simulink model "SecRwRtStRclCmdSrvCal"  (R2018b)
settings: Solver=FixedStepDiscrete  StartTime=0.0  StopTime=10.0  FixedStep=0.01  RelTol=1e-3
undefined symbols (not defined in the file or in its folder): KeSMSwPosInvalidVal_Val, PowerMode1
settings Model: Creator=sn2xws  LastModifiedBy=sn2xws
settings Model: ModifiedHistory=|
  | 2024.5.6
  | 557 新增零重力电机
settings DataIOCC: SaveFormat=StructureWithTime
settings OptimizationCC: DefaultParameterBehavior=Inlined  EnhancedBackFolding=on  PassReuseOutputArgsAs=Individual arguments  ZeroExternalMemoryAtStartup=off  ZeroInternalMemoryAtStartup=off  OptimizeBlockOrder=speed  DifferentSizesBufferReuse=on  OptimizationCustomize=off
settings DebuggingCC: ParameterTunabilityLossMsg=error
settings ModelReferenceCC: ModelReferenceNumInstancesAllowed=Single
settings SFSimCC: MATLABDynamicMemAlloc=off
settings RTWCC: SystemTargetFile=autosar.tlc  GenCodeOnly=on  TemplateMakefile=ert_default_tmf  Description=AUTOSAR  GenerateReport=on  IncludeHyperlinkInReport=on  LaunchReport=on  GenerateTraceInfo=on  GenerateTraceReport=on  GenerateTraceReportSl=on  GenerateTraceReportSf=on  GenerateTraceReportEml=on  GenerateCodeMetricsReport=on
settings CodeAppCC: ForceParamTrailComments=on  IgnoreCustomStorageClasses=off  OperatorAnnotations=on  SimulinkDataObjDesc=on  SFDataObjDesc=on  InsertBlockDesc=on
settings STFCustomTargetCC: TargetLangStandard=C99 (ISO)  MultiwordLength=256  ParMdlRefBuildCompliant=on  CompOptLevelCompliant=on  IncludeMdlTerminateFcn=off  CombineOutputUpdateFcns=on  SuppressErrorStatus=on  ERTCustomFileBanners=on  SupportNonFinite=off  SupportComplex=off  SupportContinuousTime=off  SupportNonInlinedSFcns=off  RemoveResetFunc=on  MATLABClassNameForMDSCustomization=Simulink.SoftwareTarget.ERTCustomization  AutosarCompliant=on  UseToolchainInfoCompliant=on  LookupTableObjectStructAxisOrder=2,1,3,4,...  LUTObjectStructOrderEvenSpacing=Size,Table,Breakpoints  SystemTargetFile=autosar.tlc
settings ERTTargetCC: TargetLangStandard=C99 (ISO)  ConcurrentExecutionCompliant=off  IncludeMdlTerminateFcn=off  SuppressErrorStatus=on  SupportNonFinite=off  SupportComplex=off  ModelStepFunctionPrototypeControlCompliant=off  CPPClassGenCompliant=off  AutosarCompliant=on  LookupTableObjectStructAxisOrder=2,1,3,4,...  LUTObjectStructOrderEvenSpacing=Size,Table,Breakpoints  InlinedParameterPlacement=NonHierarchical  ERTCustomFileTemplate=example_file_process.tlc  ERTFilePackagingFormat=Compact

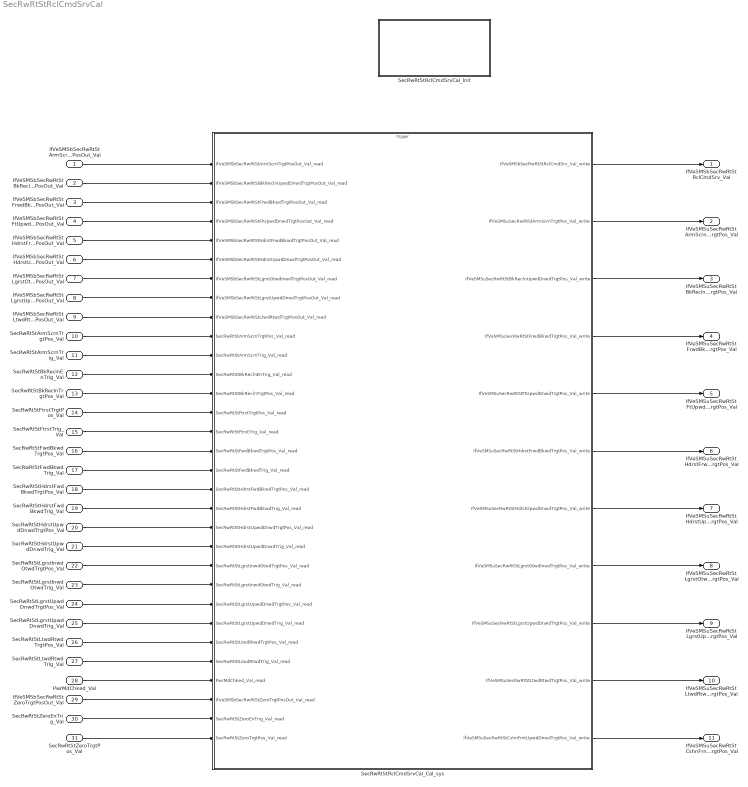
== system SecRwRtStRclCmdSrvCal ==
  IfVeSMSbSecRwRtStArmScrnTrgtPosOut_Val : Inport  OutDataTypeStr=boolean  PortDimensions=1
  IfVeSMSbSecRwRtStBkReclnUpwdDnwdTrgtPosOut_Val : Inport  Port=2  OutDataTypeStr=boolean  PortDimensions=1
  IfVeSMSbSecRwRtStFrwdBkwdTrgtPosOut_Val : Inport  Port=3  OutDataTypeStr=boolean  PortDimensions=1
  IfVeSMSbSecRwRtStFtUpwdDnwdTrgtPosOut_Val : Inport  Port=4  OutDataTypeStr=boolean  PortDimensions=1
  IfVeSMSbSecRwRtStHdrstFrwdBkwdTrgtPosOut_Val : Inport  Port=5  OutDataTypeStr=boolean  PortDimensions=1
  IfVeSMSbSecRwRtStHdrstUpwdDnwdTrgtPosOut_Val : Inport  Port=6  OutDataTypeStr=boolean  PortDimensions=1
  IfVeSMSbSecRwRtStLgrstOtwdInwdTrgtPosOut_Val : Inport  Port=7  OutDataTypeStr=boolean  PortDimensions=1
  IfVeSMSbSecRwRtStLgrstUpwdDnwdTrgtPosOut_Val : Inport  Port=8  OutDataTypeStr=boolean  PortDimensions=1
  IfVeSMSbSecRwRtStLtwdRtwdTrgtPosOut_Val : Inport  Port=9  OutDataTypeStr=boolean  PortDimensions=1
  SecRwRtStArmScrnTrgtPos_Val : Inport  Port=10  OutDataTypeStr=uint16  PortDimensions=1
  SecRwRtStArmScrnTrig_Val : Inport  Port=11  OutDataTypeStr=boolean  PortDimensions=1
  SecRwRtStBkReclnEnTrig_Val : Inport  Port=12  OutDataTypeStr=boolean  PortDimensions=1
  SecRwRtStBkReclnTrgtPos_Val : Inport  Port=13  OutDataTypeStr=uint16  PortDimensions=1
  SecRwRtStFtrstTrgtPos_Val : Inport  Port=14  OutDataTypeStr=uint16  PortDimensions=1
  SecRwRtStFtrstTrig_Val : Inport  Port=15  OutDataTypeStr=boolean  PortDimensions=1
  SecRwRtStFwdBkwdTrgtPos_Val : Inport  Port=16  OutDataTypeStr=uint16  PortDimensions=1
  SecRwRtStFwdBkwdTrig_Val : Inport  Port=17  OutDataTypeStr=boolean  PortDimensions=1
  SecRwRtStHdrstFwdBkwdTrgtPos_Val : Inport  Port=18  OutDataTypeStr=uint16  PortDimensions=1
  SecRwRtStHdrstFwdBkwdTrig_Val : Inport  Port=19  OutDataTypeStr=boolean  PortDimensions=1
  SecRwRtStHdrstUpwdDnwdTrgtPos_Val : Inport  Port=20  OutDataTypeStr=uint16  PortDimensions=1
  SecRwRtStHdrstUpwdDnwdTrig_Val : Inport  Port=21  OutDataTypeStr=boolean  PortDimensions=1
  SecRwRtStLgrstInwdOtwdTrgtPos_Val : Inport  Port=22  OutDataTypeStr=uint16  PortDimensions=1
  SecRwRtStLgrstInwdOtwdTrig_Val : Inport  Port=23  OutDataTypeStr=boolean  PortDimensions=1
  SecRwRtStLgrstUpwdDnwdTrgtPos_Val : Inport  Port=24  OutDataTypeStr=uint16  PortDimensions=1
  SecRwRtStLgrstUpwdDnwdTrig_Val : Inport  Port=25  OutDataTypeStr=boolean  PortDimensions=1
  SecRwRtStLtwdRtwdTrgtPos_Val : Inport  Port=26  OutDataTypeStr=uint16  PortDimensions=1
  SecRwRtStLtwdRtwdTrig_Val : Inport  Port=27  OutDataTypeStr=boolean  PortDimensions=1
  PwrMdChked_Val : Inport  Port=28  OutDataTypeStr=Enum: PowerMode1  PortDimensions=1
  IfVeSMSbSecRwRtStZeroTrgtPosOut_Val : Inport  Port=29  OutDataTypeStr=boolean  PortDimensions=1
  SecRwRtStZeroEnTrig_Val : Inport  Port=30  OutDataTypeStr=boolean  PortDimensions=1
  SecRwRtStZeroTrgtPos_Val : Inport  Port=31  OutDataTypeStr=uint16  PortDimensions=1
  SecRwRtStRclCmdSrvCal_Cal_sys : Subsystem
  SecRwRtStRclCmdSrvCal_Init : Subsystem
  IfVeSMSbSecRwRtStRclCmdSrv_Val : Outport  OutDataTypeStr=boolean  PortDimensions=1
  IfVeSMSuSecRwRtStArmScrnTrgtPos_Val : Outport  Port=2  OutDataTypeStr=uint16  PortDimensions=1
  IfVeSMSuSecRwRtStBkReclnUpwdDnwdTrgtPos_Val : Outport  Port=3  OutDataTypeStr=uint16  PortDimensions=1
  IfVeSMSuSecRwRtStFrwdBkwdTrgtPos_Val : Outport  Port=4  OutDataTypeStr=uint16  PortDimensions=1
  IfVeSMSuSecRwRtStFtUpwdDnwdTrgtPos_Val : Outport  Port=5  OutDataTypeStr=uint16  PortDimensions=1
  IfVeSMSuSecRwRtStHdrstFrwdBkwdTrgtPos_Val : Outport  Port=6  OutDataTypeStr=uint16  PortDimensions=1
  IfVeSMSuSecRwRtStHdrstUpwdDnwdTrgtPos_Val : Outport  Port=7  OutDataTypeStr=uint16  PortDimensions=1
  IfVeSMSuSecRwRtStLgrstOtwdInwdTrgtPos_Val : Outport  Port=8  OutDataTypeStr=uint16  PortDimensions=1
  IfVeSMSuSecRwRtStLgrstUpwdDnwdTrgtPos_Val : Outport  Port=9  OutDataTypeStr=uint16  PortDimensions=1
  IfVeSMSuSecRwRtStLtwdRtwdTrgtPos_Val : Outport  Port=10  OutDataTypeStr=uint16  PortDimensions=1
  IfVeSMSuSecRwRtStCshnFrntUpwdDnwdTrgtPos_Val : Outport  Port=11  OutDataTypeStr=uint16  PortDimensions=1
  wires:
  IfVeSMSbSecRwRtStArmScrnTrgtPosOut_Val/1 -> SecRwRtStRclCmdSrvCal_Cal_sys/1(IfVeSMSbSecRwRtStArmScrnTrgtPosOut_Val_read)
  IfVeSMSbSecRwRtStBkReclnUpwdDnwdTrgtPosOut_Val/1 -> SecRwRtStRclCmdSrvCal_Cal_sys/2(IfVeSMSbSecRwRtStBkReclnUpwdDnwdTrgtPosOut_Val_read)
  IfVeSMSbSecRwRtStFrwdBkwdTrgtPosOut_Val/1 -> SecRwRtStRclCmdSrvCal_Cal_sys/3(IfVeSMSbSecRwRtStFrwdBkwdTrgtPosOut_Val_read)
  IfVeSMSbSecRwRtStFtUpwdDnwdTrgtPosOut_Val/1 -> SecRwRtStRclCmdSrvCal_Cal_sys/4(IfVeSMSbSecRwRtStFtUpwdDnwdTrgtPosOut_Val_read)
  IfVeSMSbSecRwRtStHdrstFrwdBkwdTrgtPosOut_Val/1 -> SecRwRtStRclCmdSrvCal_Cal_sys/5(IfVeSMSbSecRwRtStHdrstFrwdBkwdTrgtPosOut_Val_read)
  IfVeSMSbSecRwRtStHdrstUpwdDnwdTrgtPosOut_Val/1 -> SecRwRtStRclCmdSrvCal_Cal_sys/6(IfVeSMSbSecRwRtStHdrstUpwdDnwdTrgtPosOut_Val_read)
  IfVeSMSbSecRwRtStLgrstOtwdInwdTrgtPosOut_Val/1 -> SecRwRtStRclCmdSrvCal_Cal_sys/7(IfVeSMSbSecRwRtStLgrstOtwdInwdTrgtPosOut_Val_read)
  IfVeSMSbSecRwRtStLgrstUpwdDnwdTrgtPosOut_Val/1 -> SecRwRtStRclCmdSrvCal_Cal_sys/8(IfVeSMSbSecRwRtStLgrstUpwdDnwdTrgtPosOut_Val_read)
  IfVeSMSbSecRwRtStLtwdRtwdTrgtPosOut_Val/1 -> SecRwRtStRclCmdSrvCal_Cal_sys/9(IfVeSMSbSecRwRtStLtwdRtwdTrgtPosOut_Val_read)
  SecRwRtStArmScrnTrgtPos_Val/1 -> SecRwRtStRclCmdSrvCal_Cal_sys/10(SecRwRtStArmScrnTrgtPos_Val_read)
  SecRwRtStArmScrnTrig_Val/1 -> SecRwRtStRclCmdSrvCal_Cal_sys/11(SecRwRtStArmScrnTrig_Val_read)
  SecRwRtStBkReclnEnTrig_Val/1 -> SecRwRtStRclCmdSrvCal_Cal_sys/12(SecRwRtStBkReclnEnTrig_Val_read)
  SecRwRtStBkReclnTrgtPos_Val/1 -> SecRwRtStRclCmdSrvCal_Cal_sys/13(SecRwRtStBkReclnTrgtPos_Val_read)
  SecRwRtStFtrstTrgtPos_Val/1 -> SecRwRtStRclCmdSrvCal_Cal_sys/14(SecRwRtStFtrstTrgtPos_Val_read)
  SecRwRtStFtrstTrig_Val/1 -> SecRwRtStRclCmdSrvCal_Cal_sys/15(SecRwRtStFtrstTrig_Val_read)
  SecRwRtStFwdBkwdTrgtPos_Val/1 -> SecRwRtStRclCmdSrvCal_Cal_sys/16(SecRwRtStFwdBkwdTrgtPos_Val_read)
  SecRwRtStFwdBkwdTrig_Val/1 -> SecRwRtStRclCmdSrvCal_Cal_sys/17(SecRwRtStFwdBkwdTrig_Val_read)
  SecRwRtStHdrstFwdBkwdTrgtPos_Val/1 -> SecRwRtStRclCmdSrvCal_Cal_sys/18(SecRwRtStHdrstFwdBkwdTrgtPos_Val_read)
  SecRwRtStHdrstFwdBkwdTrig_Val/1 -> SecRwRtStRclCmdSrvCal_Cal_sys/19(SecRwRtStHdrstFwdBkwdTrig_Val_read)
  SecRwRtStHdrstUpwdDnwdTrgtPos_Val/1 -> SecRwRtStRclCmdSrvCal_Cal_sys/20(SecRwRtStHdrstUpwdDnwdTrgtPos_Val_read)
  SecRwRtStHdrstUpwdDnwdTrig_Val/1 -> SecRwRtStRclCmdSrvCal_Cal_sys/21(SecRwRtStHdrstUpwdDnwdTrig_Val_read)
  SecRwRtStLgrstInwdOtwdTrgtPos_Val/1 -> SecRwRtStRclCmdSrvCal_Cal_sys/22(SecRwRtStLgrstInwdOtwdTrgtPos_Val_read)
  SecRwRtStLgrstInwdOtwdTrig_Val/1 -> SecRwRtStRclCmdSrvCal_Cal_sys/23(SecRwRtStLgrstInwdOtwdTrig_Val_read)
  SecRwRtStLgrstUpwdDnwdTrgtPos_Val/1 -> SecRwRtStRclCmdSrvCal_Cal_sys/24(SecRwRtStLgrstUpwdDnwdTrgtPos_Val_read)
  SecRwRtStLgrstUpwdDnwdTrig_Val/1 -> SecRwRtStRclCmdSrvCal_Cal_sys/25(SecRwRtStLgrstUpwdDnwdTrig_Val_read)
  SecRwRtStLtwdRtwdTrgtPos_Val/1 -> SecRwRtStRclCmdSrvCal_Cal_sys/26(SecRwRtStLtwdRtwdTrgtPos_Val_read)
  SecRwRtStLtwdRtwdTrig_Val/1 -> SecRwRtStRclCmdSrvCal_Cal_sys/27(SecRwRtStLtwdRtwdTrig_Val_read)
  SecRwRtStRclCmdSrvCal_Cal_sys/1(IfVeSMSbSecRwRtStRclCmdSrv_Val_write) -> IfVeSMSbSecRwRtStRclCmdSrv_Val/1
  SecRwRtStRclCmdSrvCal_Cal_sys/2(IfVeSMSuSecRwRtStArmScrnTrgtPos_Val_write) -> IfVeSMSuSecRwRtStArmScrnTrgtPos_Val/1
  SecRwRtStRclCmdSrvCal_Cal_sys/3(IfVeSMSuSecRwRtStBkReclnUpwdDnwdTrgtPos_Val_write) -> IfVeSMSuSecRwRtStBkReclnUpwdDnwdTrgtPos_Val/1
  SecRwRtStRclCmdSrvCal_Cal_sys/4(IfVeSMSuSecRwRtStFrwdBkwdTrgtPos_Val_write) -> IfVeSMSuSecRwRtStFrwdBkwdTrgtPos_Val/1
  SecRwRtStRclCmdSrvCal_Cal_sys/5(IfVeSMSuSecRwRtStFtUpwdDnwdTrgtPos_Val_write) -> IfVeSMSuSecRwRtStFtUpwdDnwdTrgtPos_Val/1
  SecRwRtStRclCmdSrvCal_Cal_sys/6(IfVeSMSuSecRwRtStHdrstFrwdBkwdTrgtPos_Val_write) -> IfVeSMSuSecRwRtStHdrstFrwdBkwdTrgtPos_Val/1
  SecRwRtStRclCmdSrvCal_Cal_sys/7(IfVeSMSuSecRwRtStHdrstUpwdDnwdTrgtPos_Val_write) -> IfVeSMSuSecRwRtStHdrstUpwdDnwdTrgtPos_Val/1
  SecRwRtStRclCmdSrvCal_Cal_sys/8(IfVeSMSuSecRwRtStLgrstOtwdInwdTrgtPos_Val_write) -> IfVeSMSuSecRwRtStLgrstOtwdInwdTrgtPos_Val/1
  SecRwRtStRclCmdSrvCal_Cal_sys/9(IfVeSMSuSecRwRtStLgrstUpwdDnwdTrgtPos_Val_write) -> IfVeSMSuSecRwRtStLgrstUpwdDnwdTrgtPos_Val/1
  SecRwRtStRclCmdSrvCal_Cal_sys/10(IfVeSMSuSecRwRtStLtwdRtwdTrgtPos_Val_write) -> IfVeSMSuSecRwRtStLtwdRtwdTrgtPos_Val/1
  PwrMdChked_Val/1 -> SecRwRtStRclCmdSrvCal_Cal_sys/28(PwrMdChked_Val_read)
  IfVeSMSbSecRwRtStZeroTrgtPosOut_Val/1 -> SecRwRtStRclCmdSrvCal_Cal_sys/29(IfVeSMSbSecRwRtStZeroTrgtPosOut_Val_read)
  SecRwRtStZeroEnTrig_Val/1 -> SecRwRtStRclCmdSrvCal_Cal_sys/30(SecRwRtStZeroEnTrig_Val_read)
  SecRwRtStZeroTrgtPos_Val/1 -> SecRwRtStRclCmdSrvCal_Cal_sys/31(SecRwRtStZeroTrgtPos_Val_read)
  SecRwRtStRclCmdSrvCal_Cal_sys/11(IfVeSMSuSecRwRtStCshnFrntUpwdDnwdTrgtPos_Val_write) -> IfVeSMSuSecRwRtStCshnFrntUpwdDnwdTrgtPos_Val/1

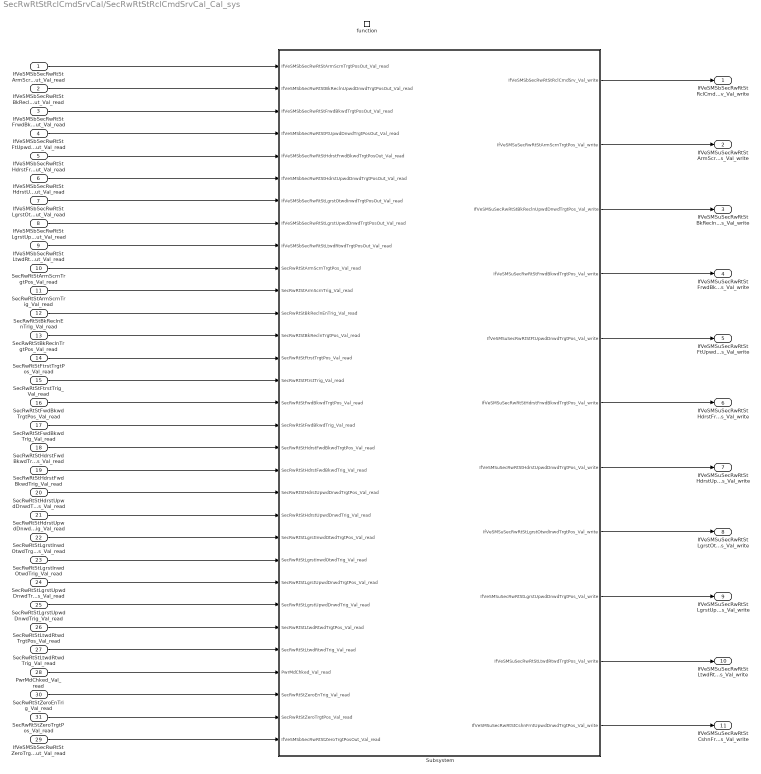
== system SecRwRtStRclCmdSrvCal/SecRwRtStRclCmdSrvCal_Cal_sys ==
  IfVeSMSbSecRwRtStArmScrnTrgtPosOut_Val_read : Inport
  IfVeSMSbSecRwRtStBkReclnUpwdDnwdTrgtPosOut_Val_read : Inport  Port=2
  IfVeSMSbSecRwRtStFrwdBkwdTrgtPosOut_Val_read : Inport  Port=3
  IfVeSMSbSecRwRtStFtUpwdDnwdTrgtPosOut_Val_read : Inport  Port=4
  IfVeSMSbSecRwRtStHdrstFrwdBkwdTrgtPosOut_Val_read : Inport  Port=5
  IfVeSMSbSecRwRtStHdrstUpwdDnwdTrgtPosOut_Val_read : Inport  Port=6
  IfVeSMSbSecRwRtStLgrstOtwdInwdTrgtPosOut_Val_read : Inport  Port=7
  IfVeSMSbSecRwRtStLgrstUpwdDnwdTrgtPosOut_Val_read : Inport  Port=8
  IfVeSMSbSecRwRtStLtwdRtwdTrgtPosOut_Val_read : Inport  Port=9
  SecRwRtStArmScrnTrgtPos_Val_read : Inport  Port=10
  SecRwRtStArmScrnTrig_Val_read : Inport  Port=11
  SecRwRtStBkReclnEnTrig_Val_read : Inport  Port=12
  SecRwRtStBkReclnTrgtPos_Val_read : Inport  Port=13
  SecRwRtStFtrstTrgtPos_Val_read : Inport  Port=14
  SecRwRtStFtrstTrig_Val_read : Inport  Port=15
  SecRwRtStFwdBkwdTrgtPos_Val_read : Inport  Port=16
  SecRwRtStFwdBkwdTrig_Val_read : Inport  Port=17
  SecRwRtStHdrstFwdBkwdTrgtPos_Val_read : Inport  Port=18
  SecRwRtStHdrstFwdBkwdTrig_Val_read : Inport  Port=19
  SecRwRtStHdrstUpwdDnwdTrgtPos_Val_read : Inport  Port=20
  SecRwRtStHdrstUpwdDnwdTrig_Val_read : Inport  Port=21
  SecRwRtStLgrstInwdOtwdTrgtPos_Val_read : Inport  Port=22
  SecRwRtStLgrstInwdOtwdTrig_Val_read : Inport  Port=23
  SecRwRtStLgrstUpwdDnwdTrgtPos_Val_read : Inport  Port=24
  SecRwRtStLgrstUpwdDnwdTrig_Val_read : Inport  Port=25
  SecRwRtStLtwdRtwdTrgtPos_Val_read : Inport  Port=26
  SecRwRtStLtwdRtwdTrig_Val_read : Inport  Port=27
  PwrMdChked_Val_read : Inport  Port=28
  IfVeSMSbSecRwRtStZeroTrgtPosOut_Val_read : Inport  Port=29
  SecRwRtStZeroEnTrig_Val_read : Inport  Port=30
  SecRwRtStZeroTrgtPos_Val_read : Inport  Port=31
  function : TriggerPort  TriggerType=function-call  IsSimulinkFunction=on  FunctionName=SecRwRtStRclCmdSrvCal_Cal  VariantControl=(inherit)
  Subsystem : Subsystem
  IfVeSMSbSecRwRtStRclCmdSrv_Val_write : Outport
      settings: EnsureOutportIsVirtual=on
  IfVeSMSuSecRwRtStArmScrnTrgtPos_Val_write : Outport  Port=2
      settings: EnsureOutportIsVirtual=on
  IfVeSMSuSecRwRtStBkReclnUpwdDnwdTrgtPos_Val_write : Outport  Port=3
      settings: EnsureOutportIsVirtual=on
  IfVeSMSuSecRwRtStFrwdBkwdTrgtPos_Val_write : Outport  Port=4
      settings: EnsureOutportIsVirtual=on
  IfVeSMSuSecRwRtStFtUpwdDnwdTrgtPos_Val_write : Outport  Port=5
      settings: EnsureOutportIsVirtual=on
  IfVeSMSuSecRwRtStHdrstFrwdBkwdTrgtPos_Val_write : Outport  Port=6
      settings: EnsureOutportIsVirtual=on
  IfVeSMSuSecRwRtStHdrstUpwdDnwdTrgtPos_Val_write : Outport  Port=7
      settings: EnsureOutportIsVirtual=on
  IfVeSMSuSecRwRtStLgrstOtwdInwdTrgtPos_Val_write : Outport  Port=8
      settings: EnsureOutportIsVirtual=on
  IfVeSMSuSecRwRtStLgrstUpwdDnwdTrgtPos_Val_write : Outport  Port=9
      settings: EnsureOutportIsVirtual=on
  IfVeSMSuSecRwRtStLtwdRtwdTrgtPos_Val_write : Outport  Port=10
      settings: EnsureOutportIsVirtual=on
  IfVeSMSuSecRwRtStCshnFrntUpwdDnwdTrgtPos_Val_write : Outport  Port=11
      settings: EnsureOutportIsVirtual=on
  wires:
  SecRwRtStFwdBkwdTrgtPos_Val_read/1 -> Subsystem/16(SecRwRtStFwdBkwdTrgtPos_Val_read)
  SecRwRtStFwdBkwdTrig_Val_read/1 -> Subsystem/17(SecRwRtStFwdBkwdTrig_Val_read)
  SecRwRtStHdrstFwdBkwdTrgtPos_Val_read/1 -> Subsystem/18(SecRwRtStHdrstFwdBkwdTrgtPos_Val_read)
  SecRwRtStFtrstTrgtPos_Val_read/1 -> Subsystem/14(SecRwRtStFtrstTrgtPos_Val_read)
  SecRwRtStFtrstTrig_Val_read/1 -> Subsystem/15(SecRwRtStFtrstTrig_Val_read)
  SecRwRtStHdrstFwdBkwdTrig_Val_read/1 -> Subsystem/19(SecRwRtStHdrstFwdBkwdTrig_Val_read)
  SecRwRtStHdrstUpwdDnwdTrgtPos_Val_read/1 -> Subsystem/20(SecRwRtStHdrstUpwdDnwdTrgtPos_Val_read)
  SecRwRtStArmScrnTrig_Val_read/1 -> Subsystem/11(SecRwRtStArmScrnTrig_Val_read)
  SecRwRtStBkReclnEnTrig_Val_read/1 -> Subsystem/12(SecRwRtStBkReclnEnTrig_Val_read)
  SecRwRtStBkReclnTrgtPos_Val_read/1 -> Subsystem/13(SecRwRtStBkReclnTrgtPos_Val_read)
  SecRwRtStHdrstUpwdDnwdTrig_Val_read/1 -> Subsystem/21(SecRwRtStHdrstUpwdDnwdTrig_Val_read)
  SecRwRtStLgrstInwdOtwdTrgtPos_Val_read/1 -> Subsystem/22(SecRwRtStLgrstInwdOtwdTrgtPos_Val_read)
  SecRwRtStLgrstInwdOtwdTrig_Val_read/1 -> Subsystem/23(SecRwRtStLgrstInwdOtwdTrig_Val_read)
  IfVeSMSbSecRwRtStLtwdRtwdTrgtPosOut_Val_read/1 -> Subsystem/9(IfVeSMSbSecRwRtStLtwdRtwdTrgtPosOut_Val_read)
  SecRwRtStArmScrnTrgtPos_Val_read/1 -> Subsystem/10(SecRwRtStArmScrnTrgtPos_Val_read)
  SecRwRtStLgrstUpwdDnwdTrgtPos_Val_read/1 -> Subsystem/24(SecRwRtStLgrstUpwdDnwdTrgtPos_Val_read)
  SecRwRtStLgrstUpwdDnwdTrig_Val_read/1 -> Subsystem/25(SecRwRtStLgrstUpwdDnwdTrig_Val_read)
  IfVeSMSbSecRwRtStHdrstUpwdDnwdTrgtPosOut_Val_read/1 -> Subsystem/6(IfVeSMSbSecRwRtStHdrstUpwdDnwdTrgtPosOut_Val_read)
  IfVeSMSbSecRwRtStLgrstOtwdInwdTrgtPosOut_Val_read/1 -> Subsystem/7(IfVeSMSbSecRwRtStLgrstOtwdInwdTrgtPosOut_Val_read)
  IfVeSMSbSecRwRtStLgrstUpwdDnwdTrgtPosOut_Val_read/1 -> Subsystem/8(IfVeSMSbSecRwRtStLgrstUpwdDnwdTrgtPosOut_Val_read)
  SecRwRtStLtwdRtwdTrgtPos_Val_read/1 -> Subsystem/26(SecRwRtStLtwdRtwdTrgtPos_Val_read)
  SecRwRtStLtwdRtwdTrig_Val_read/1 -> Subsystem/27(SecRwRtStLtwdRtwdTrig_Val_read)
  IfVeSMSbSecRwRtStFtUpwdDnwdTrgtPosOut_Val_read/1 -> Subsystem/4(IfVeSMSbSecRwRtStFtUpwdDnwdTrgtPosOut_Val_read)
  IfVeSMSbSecRwRtStHdrstFrwdBkwdTrgtPosOut_Val_read/1 -> Subsystem/5(IfVeSMSbSecRwRtStHdrstFrwdBkwdTrgtPosOut_Val_read)
  IfVeSMSbSecRwRtStArmScrnTrgtPosOut_Val_read/1 -> Subsystem/1(IfVeSMSbSecRwRtStArmScrnTrgtPosOut_Val_read)
  IfVeSMSbSecRwRtStBkReclnUpwdDnwdTrgtPosOut_Val_read/1 -> Subsystem/2(IfVeSMSbSecRwRtStBkReclnUpwdDnwdTrgtPosOut_Val_read)
  IfVeSMSbSecRwRtStFrwdBkwdTrgtPosOut_Val_read/1 -> Subsystem/3(IfVeSMSbSecRwRtStFrwdBkwdTrgtPosOut_Val_read)
  Subsystem/1(IfVeSMSbSecRwRtStRclCmdSrv_Val_write) -> IfVeSMSbSecRwRtStRclCmdSrv_Val_write/1
  Subsystem/2(IfVeSMSuSecRwRtStArmScrnTrgtPos_Val_write) -> IfVeSMSuSecRwRtStArmScrnTrgtPos_Val_write/1
  Subsystem/3(IfVeSMSuSecRwRtStBkReclnUpwdDnwdTrgtPos_Val_write) -> IfVeSMSuSecRwRtStBkReclnUpwdDnwdTrgtPos_Val_write/1
  Subsystem/4(IfVeSMSuSecRwRtStFrwdBkwdTrgtPos_Val_write) -> IfVeSMSuSecRwRtStFrwdBkwdTrgtPos_Val_write/1
  Subsystem/5(IfVeSMSuSecRwRtStFtUpwdDnwdTrgtPos_Val_write) -> IfVeSMSuSecRwRtStFtUpwdDnwdTrgtPos_Val_write/1
  Subsystem/6(IfVeSMSuSecRwRtStHdrstFrwdBkwdTrgtPos_Val_write) -> IfVeSMSuSecRwRtStHdrstFrwdBkwdTrgtPos_Val_write/1
  Subsystem/7(IfVeSMSuSecRwRtStHdrstUpwdDnwdTrgtPos_Val_write) -> IfVeSMSuSecRwRtStHdrstUpwdDnwdTrgtPos_Val_write/1
  Subsystem/8(IfVeSMSuSecRwRtStLgrstOtwdInwdTrgtPos_Val_write) -> IfVeSMSuSecRwRtStLgrstOtwdInwdTrgtPos_Val_write/1
  Subsystem/9(IfVeSMSuSecRwRtStLgrstUpwdDnwdTrgtPos_Val_write) -> IfVeSMSuSecRwRtStLgrstUpwdDnwdTrgtPos_Val_write/1
  Subsystem/10(IfVeSMSuSecRwRtStLtwdRtwdTrgtPos_Val_write) -> IfVeSMSuSecRwRtStLtwdRtwdTrgtPos_Val_write/1
  PwrMdChked_Val_read/1 -> Subsystem/28(PwrMdChked_Val_read)
  IfVeSMSbSecRwRtStZeroTrgtPosOut_Val_read/1 -> Subsystem/31(IfVeSMSbSecRwRtStZeroTrgtPosOut_Val_read)
  Subsystem/11(IfVeSMSuSecRwRtStCshnFrntUpwdDnwdTrgtPos_Val_write) -> IfVeSMSuSecRwRtStCshnFrntUpwdDnwdTrgtPos_Val_write/1
  SecRwRtStZeroEnTrig_Val_read/1 -> Subsystem/29(SecRwRtStZeroEnTrig_Val_read)
  SecRwRtStZeroTrgtPos_Val_read/1 -> Subsystem/30(SecRwRtStZeroTrgtPos_Val_read)

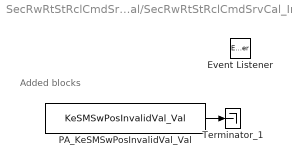
== system SecRwRtStRclCmdSrvCal/SecRwRtStRclCmdSrvCal_Init ==
  note: Added blocks
  Event Listener : EventListener  EventName=reset
  PA_KeSMSwPosInvalidVal_Val : Constant  Value=KeSMSwPosInvalidVal_Val
  Terminator_1 : Terminator
  wires:
  PA_KeSMSwPosInvalidVal_Val/1 -> Terminator_1/1

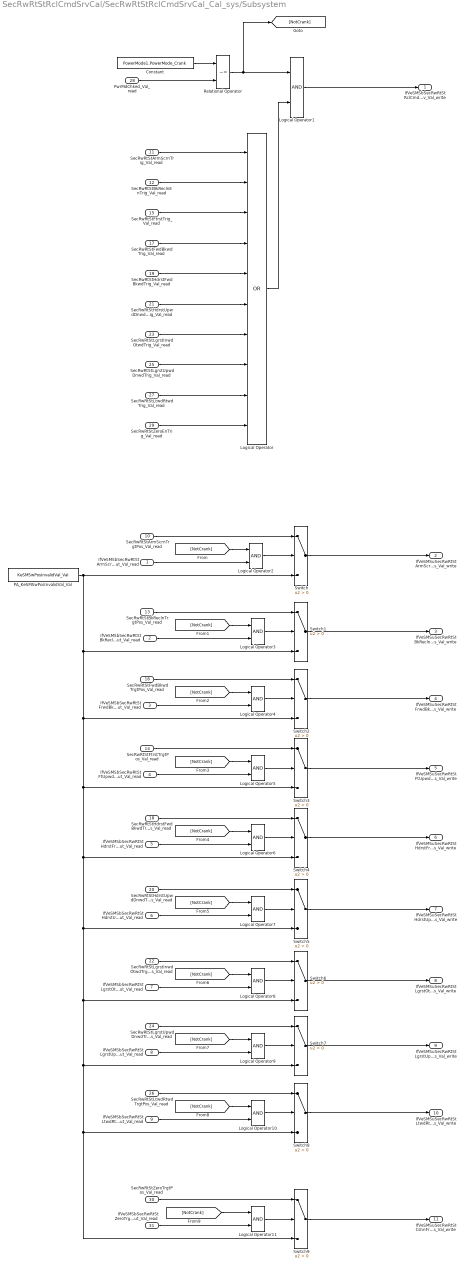
== system SecRwRtStRclCmdSrvCal/SecRwRtStRclCmdSrvCal_Cal_sys/Subsystem ==
  IfVeSMSbSecRwRtStArmScrnTrgtPosOut_Val_read : Inport
  IfVeSMSbSecRwRtStBkReclnUpwdDnwdTrgtPosOut_Val_read : Inport  Port=2
  IfVeSMSbSecRwRtStFrwdBkwdTrgtPosOut_Val_read : Inport  Port=3
  IfVeSMSbSecRwRtStFtUpwdDnwdTrgtPosOut_Val_read : Inport  Port=4
  IfVeSMSbSecRwRtStHdrstFrwdBkwdTrgtPosOut_Val_read : Inport  Port=5
  IfVeSMSbSecRwRtStHdrstUpwdDnwdTrgtPosOut_Val_read : Inport  Port=6
  IfVeSMSbSecRwRtStLgrstOtwdInwdTrgtPosOut_Val_read : Inport  Port=7
  IfVeSMSbSecRwRtStLgrstUpwdDnwdTrgtPosOut_Val_read : Inport  Port=8
  IfVeSMSbSecRwRtStLtwdRtwdTrgtPosOut_Val_read : Inport  Port=9
  SecRwRtStArmScrnTrgtPos_Val_read : Inport  Port=10
  SecRwRtStArmScrnTrig_Val_read : Inport  Port=11
  SecRwRtStBkReclnEnTrig_Val_read : Inport  Port=12
  SecRwRtStBkReclnTrgtPos_Val_read : Inport  Port=13
  SecRwRtStFtrstTrgtPos_Val_read : Inport  Port=14
  SecRwRtStFtrstTrig_Val_read : Inport  Port=15
  SecRwRtStFwdBkwdTrgtPos_Val_read : Inport  Port=16
  SecRwRtStFwdBkwdTrig_Val_read : Inport  Port=17
  SecRwRtStHdrstFwdBkwdTrgtPos_Val_read : Inport  Port=18
  SecRwRtStHdrstFwdBkwdTrig_Val_read : Inport  Port=19
  SecRwRtStHdrstUpwdDnwdTrgtPos_Val_read : Inport  Port=20
  SecRwRtStHdrstUpwdDnwdTrig_Val_read : Inport  Port=21
  SecRwRtStLgrstInwdOtwdTrgtPos_Val_read : Inport  Port=22
  SecRwRtStLgrstInwdOtwdTrig_Val_read : Inport  Port=23
  SecRwRtStLgrstUpwdDnwdTrgtPos_Val_read : Inport  Port=24
  SecRwRtStLgrstUpwdDnwdTrig_Val_read : Inport  Port=25
  SecRwRtStLtwdRtwdTrgtPos_Val_read : Inport  Port=26
  SecRwRtStLtwdRtwdTrig_Val_read : Inport  Port=27
  PwrMdChked_Val_read : Inport  Port=28
  SecRwRtStZeroEnTrig_Val_read : Inport  Port=29
  SecRwRtStZeroTrgtPos_Val_read : Inport  Port=30
  IfVeSMSbSecRwRtStZeroTrgtPosOut_Val_read : Inport  Port=31
  Constant : Constant  Value=PowerMode1.PowerMode_Crank  OutDataTypeStr=Enum: PowerMode1
  Logical Operator : Logic  Operator=OR  Inputs=10  AllPortsSameDT=off  OutDataTypeStr=boolean
  Logical Operator{1..11} (11 alike) : Logic  AllPortsSameDT=off  OutDataTypeStr=boolean
  PA_KeSMSwPosInvalidVal_Val : Constant  Value=KeSMSwPosInvalidVal_Val
  Relational Operator : RelationalOperator  Operator=~=  OutDataTypeStr=boolean  RndMeth=Simplest
  Switch{,1..9} (10 alike) : Switch  Criteria=u2 > Threshold
  IfVeSMSbSecRwRtStRclCmdSrv_Val_write : Outport
      settings: EnsureOutportIsVirtual=on
  IfVeSMSuSecRwRtStArmScrnTrgtPos_Val_write : Outport  Port=2
      settings: EnsureOutportIsVirtual=on
  IfVeSMSuSecRwRtStBkReclnUpwdDnwdTrgtPos_Val_write : Outport  Port=3
      settings: EnsureOutportIsVirtual=on
  IfVeSMSuSecRwRtStFrwdBkwdTrgtPos_Val_write : Outport  Port=4
      settings: EnsureOutportIsVirtual=on
  IfVeSMSuSecRwRtStFtUpwdDnwdTrgtPos_Val_write : Outport  Port=5
      settings: EnsureOutportIsVirtual=on
  IfVeSMSuSecRwRtStHdrstFrwdBkwdTrgtPos_Val_write : Outport  Port=6
      settings: EnsureOutportIsVirtual=on
  IfVeSMSuSecRwRtStHdrstUpwdDnwdTrgtPos_Val_write : Outport  Port=7
      settings: EnsureOutportIsVirtual=on
  IfVeSMSuSecRwRtStLgrstOtwdInwdTrgtPos_Val_write : Outport  Port=8
      settings: EnsureOutportIsVirtual=on
  IfVeSMSuSecRwRtStLgrstUpwdDnwdTrgtPos_Val_write : Outport  Port=9
      settings: EnsureOutportIsVirtual=on
  IfVeSMSuSecRwRtStLtwdRtwdTrgtPos_Val_write : Outport  Port=10
      settings: EnsureOutportIsVirtual=on
  IfVeSMSuSecRwRtStCshnFrntUpwdDnwdTrgtPos_Val_write : Outport  Port=11
      settings: EnsureOutportIsVirtual=on
  wires:
  SecRwRtStArmScrnTrig_Val_read/1 -> Logical Operator/1
  SecRwRtStFwdBkwdTrig_Val_read/1 -> Logical Operator/4
  SecRwRtStBkReclnTrgtPos_Val_read/1 -> Switch1/1
  PA_KeSMSwPosInvalidVal_Val/1 -> Switch2/3, Switch9/3, Switch8/3, Switch7/3, Switch6/3, Switch5/3, Switch4/3, Switch3/3, Switch1/3, Switch/3
  SecRwRtStLgrstUpwdDnwdTrig_Val_read/1 -> Logical Operator/8
  Switch1/1 -> IfVeSMSuSecRwRtStBkReclnUpwdDnwdTrgtPos_Val_write/1
  Switch3/1 -> IfVeSMSuSecRwRtStFtUpwdDnwdTrgtPos_Val_write/1
  SecRwRtStLtwdRtwdTrig_Val_read/1 -> Logical Operator/9
  SecRwRtStFtrstTrgtPos_Val_read/1 -> Switch3/1
  Switch4/1 -> IfVeSMSuSecRwRtStHdrstFrwdBkwdTrgtPos_Val_write/1
  SecRwRtStFtrstTrig_Val_read/1 -> Logical Operator/3
  SecRwRtStHdrstUpwdDnwdTrgtPos_Val_read/1 -> Switch5/1
  Switch2/1 -> IfVeSMSuSecRwRtStFrwdBkwdTrgtPos_Val_write/1
  SecRwRtStArmScrnTrgtPos_Val_read/1 -> Switch/1
  Switch/1 -> IfVeSMSuSecRwRtStArmScrnTrgtPos_Val_write/1
  SecRwRtStHdrstFwdBkwdTrgtPos_Val_read/1 -> Switch4/1
  SecRwRtStLtwdRtwdTrgtPos_Val_read/1 -> Switch8/1
  SecRwRtStLgrstUpwdDnwdTrgtPos_Val_read/1 -> Switch7/1
  Switch5/1 -> IfVeSMSuSecRwRtStHdrstUpwdDnwdTrgtPos_Val_write/1
  Switch6/1 -> IfVeSMSuSecRwRtStLgrstOtwdInwdTrgtPos_Val_write/1
  SecRwRtStLgrstInwdOtwdTrgtPos_Val_read/1 -> Switch6/1
  SecRwRtStFwdBkwdTrgtPos_Val_read/1 -> Switch2/1
  Switch8/1 -> IfVeSMSuSecRwRtStLtwdRtwdTrgtPos_Val_write/1
  SecRwRtStLgrstInwdOtwdTrig_Val_read/1 -> Logical Operator/7
  SecRwRtStHdrstFwdBkwdTrig_Val_read/1 -> Logical Operator/5
  Switch7/1 -> IfVeSMSuSecRwRtStLgrstUpwdDnwdTrgtPos_Val_write/1
  SecRwRtStHdrstUpwdDnwdTrig_Val_read/1 -> Logical Operator/6
  SecRwRtStBkReclnEnTrig_Val_read/1 -> Logical Operator/2
  PwrMdChked_Val_read/1 -> Relational Operator/2
  Relational Operator/1 -> [NotCrank], Logical Operator1/1
  Logical Operator1/1 -> IfVeSMSbSecRwRtStRclCmdSrv_Val_write/1
  Constant/1 -> Relational Operator/1
  Logical Operator/1 -> Logical Operator1/2
  Logical Operator2/1 -> Switch/2
  IfVeSMSbSecRwRtStArmScrnTrgtPosOut_Val_read/1 -> Logical Operator2/2
  [NotCrank] -> Logical Operator2/1
  [NotCrank] -> Logical Operator3/1
  IfVeSMSbSecRwRtStBkReclnUpwdDnwdTrgtPosOut_Val_read/1 -> Logical Operator3/2
  Logical Operator3/1 -> Switch1/2
  Logical Operator4/1 -> Switch2/2
  IfVeSMSbSecRwRtStFrwdBkwdTrgtPosOut_Val_read/1 -> Logical Operator4/2
  [NotCrank] -> Logical Operator4/1
  [NotCrank] -> Logical Operator5/1
  IfVeSMSbSecRwRtStFtUpwdDnwdTrgtPosOut_Val_read/1 -> Logical Operator5/2
  Logical Operator5/1 -> Switch3/2
  Logical Operator6/1 -> Switch4/2
  IfVeSMSbSecRwRtStHdrstFrwdBkwdTrgtPosOut_Val_read/1 -> Logical Operator6/2
  [NotCrank] -> Logical Operator6/1
  [NotCrank] -> Logical Operator7/1
  IfVeSMSbSecRwRtStHdrstUpwdDnwdTrgtPosOut_Val_read/1 -> Logical Operator7/2
  Logical Operator7/1 -> Switch5/2
  Logical Operator8/1 -> Switch6/2
  IfVeSMSbSecRwRtStLgrstOtwdInwdTrgtPosOut_Val_read/1 -> Logical Operator8/2
  [NotCrank] -> Logical Operator8/1
  [NotCrank] -> Logical Operator9/1
  IfVeSMSbSecRwRtStLgrstUpwdDnwdTrgtPosOut_Val_read/1 -> Logical Operator9/2
  Logical Operator9/1 -> Switch7/2
  Logical Operator10/1 -> Switch8/2
  IfVeSMSbSecRwRtStLtwdRtwdTrgtPosOut_Val_read/1 -> Logical Operator10/2
  [NotCrank] -> Logical Operator10/1
  Switch9/1 -> IfVeSMSuSecRwRtStCshnFrntUpwdDnwdTrgtPos_Val_write/1
  Logical Operator11/1 -> Switch9/2
  [NotCrank] -> Logical Operator11/1
  SecRwRtStZeroEnTrig_Val_read/1 -> Logical Operator/10
  SecRwRtStZeroTrgtPos_Val_read/1 -> Switch9/1
  IfVeSMSbSecRwRtStZeroTrgtPosOut_Val_read/1 -> Logical Operator11/2
